simulink model "sampleModel646original"  (R2021b)
settings: Solver=VariableStepAuto  StartTime=0.0  StopTime=10.0  RelTol=1e-3
undefined symbols (not defined in the file): DiscIntNeverNeededParam, Newton, Raphson, sigbuilder_block
libraries: simulink x194, slpidlib x27
(part 2 of 5)

== system sampleModel646original/emi_1101 ==
  In1 : Inport
  emi_1102 : Inport  Port=2
  emi_1104 : Sin  TimeSource=Use external signal  SampleTime=0
  emi_1105 : simulink/Discrete/Difference  ICPrevInput=0.0  OutMin=[]  OutMax=[]  OutDataType=fixdt(1, 16)  OutScaling=2^-10  DoSatur=off
  emi_1106 : Sqrt  Operator=rSqrt  SaturateOnIntegerOverflow=on
  emi_1107 : DiscreteStateSpace  SampleTime=-1
  emi_1108 : Sin  TimeSource=Use external signal  SampleTime=0
  emi_1109 : RateLimiter  SampleTimeMode=inherited
  emi_1110 : Sin  TimeSource=Use external signal  SampleTime=0
  emi_1111 : slpidlib/PID Controller  Controller=PID  Form=Parallel  TimeDomain=Discrete-time  UseExternalTs=off  SampleTime=-1  IntegratorMethod=Forward Euler  FilterMethod=Forward Euler  ControllerParametersSource=internal  P=1  I=1  D=0  UseFilter=on  N=100  TunerSelectOption=Transfer Function Based (PID Tuner App)  InitialConditionSource=internal  InitialConditionForIntegrator=0  InitialConditionForFilter=0  DifferentiatorICPrevScaledInput=0  ExternalReset=none  TrackingMode=off  Kt=1  LimitOutput=off  SatLimitsSource=internal  UpperSaturationLimit=inf  LowerSaturationLimit=-inf  LinearizeAsGain=off  AntiWindupMode=none  Kb=1  POutMin=[]  POutMax=[]  IOutMin=[]  IOutMax=[]  DOutMin=[]  DOutMax=[]  NOutMin=[]  NOutMax=[]  SumOutMin=[]  SumOutMax=[]  SaturationOutMin=[]  SaturationOutMax=[]  PParamMin=[]  PParamMax=[]  IParamMin=[]  IParamMax=[]  DParamMin=[]  DParamMax=[]  NParamMin=[]  NParamMax=[]  KbParamMin=[]  KbParamMax=[]  KtParamMin=[]  KtParamMax=[]  KbOutMin=[]  KbOutMax=[]  KtOutMin=[]  KtOutMax=[]  IntegratorOutMin=[]  IntegratorOutMax=[]  FilterOutMin=[]  FilterOutMax=[]  SumI1OutMin=[]  SumI1OutMax=[]  SumI2OutMin=[]  SumI2OutMax=[]  SumI3OutMin=[]  SumI3OutMax=[]  SumI4OutMin=[]  SumI4OutMax=[]  SumDOutMin=[]  SumDOutMax=[]  DifferentiatorOutMin=[]  DifferentiatorOutMax=[]  FilterDiffOutCoefMin=[]  FilterDiffOutCoefMax=[]  ReciprocalOutMin=[]  ReciprocalOutMax=[]  SumDenOutMin=[]  SumDenOutMax=[]  SumNumOutMin=[]  SumNumOutMax=[]  DivideOutMin=[]  DivideOutMax=[]  UdiffTsProdOutMin=[]  UdiffTsProdOutMax=[]  NTsProdOutMin=[]  NTsProdOutMax=[]  UintegralTsProdOutMin=[]  UintegralTsProdOutMax=[]  UngainTsProdOutMin=[]  UngainTsProdOutMax=[]  IntegratorContinuousStateAttributes=''  IntegratorStateMustResolveToSignalObject=off  IntegratorRTWStateStorageClass=Auto  FilterContinuousStateAttributes=''  FilterStateMustResolveToSignalObject=off  FilterRTWStateStorageClass=Auto  ParallelPVariant=InternalParameters  IdealPVariant=Disabled  IVariant=InternalParameters  DVariant=InternalParameters  IntegratorVariant=Discrete  SatVariant=Disabled  AWVariant=Passthrough  PCopyVariant=Disabled  TRVariant=Disabled  FdbkBlocksVariant=Forward  IdealPFdbkVariant=Disabled  SatFdbkVariant=Disabled  DerivativeFilterVariant=ForwardEulerFilter  NVariant=InternalParameters  NCopyVariant=Disabled  FilterICVariant=InternalICsFilter  IntegratorICVariant=InternalICs  ExternalResetVariant=Disabled  TRSumVariant=Passthrough  SumFdbkVariant=Disabled  SumVariant=Sum_PID  TsampFilterVariant=InternalTs  TsampNgainVariant=Passthrough  TsampIntegralVariant=Passthrough  ExternalSaturationOutDataTypeStr=Inherit: Same as second input
  emi_1112 : DiscreteFilter
  emi_1113 : simulink/Discrete/Transfer Fcn First Order  PoleZ=0.95  ICPrevOutput=0.0  DoSatur=off
  emi_1114 : Math  SaturateOnIntegerOverflow=on
  emi_1115 : DeadZone  SaturateOnIntegerOverflow=on
  emi_1116 : DiscreteTransferFcn
  emi_1117 : simulink/Sources/Chirp Signal  f1=0.1  T=100  f2=1
  Out1 : Outport
  emi_1103 : Outport  Port=2
  wires:
  In1/1 -> Out1/1
  emi_1104/1 -> emi_1105/1
  emi_1105/1 -> emi_1106/1
  emi_1106/1 -> emi_1107/1
  emi_1107/1 -> emi_1108/1
  emi_1108/1 -> emi_1109/1
  emi_1109/1 -> emi_1110/1
  emi_1110/1 -> emi_1111/1
  emi_1111/1 -> emi_1112/1
  emi_1112/1 -> emi_1113/1
  emi_1113/1 -> emi_1114/1
  emi_1114/1 -> emi_1115/1
  emi_1115/1 -> emi_1116/1
  emi_1117/1 -> emi_1104/1
  emi_1116/1 -> emi_1103/1

== system sampleModel646original/emi_1124 ==
  emi_1131 : Inport
  Action Port : ActionPort  ActionPortLabel=if(-1.382844e+09 > u1)
  emi_{1128..1129,1136,1138} (4 alike) : Math  SaturateOnIntegerOverflow=on
  emi_1130 : MinMax
  emi_{1133..1135,1143} (4 alike) : Sin  TimeSource=Use external signal  SampleTime=0
  emi_{1137,1139..1140,1142} (4 alike) : UnaryMinus
  emi_1141 : Sqrt  Operator=rSqrt  SaturateOnIntegerOverflow=on
  emi_1144 : Product  Inputs=*
  emi_1145 : Ground
  emi_1132 : Outport
  wires:
  emi_1131/1 -> emi_1128/1
  emi_1128/1 -> emi_1129/1
  emi_1129/1 -> emi_1130/1
  emi_1133/1 -> emi_1134/1
  emi_1134/1 -> emi_1135/1
  emi_1135/1 -> emi_1136/1
  emi_1136/1 -> emi_1137/1
  emi_1137/1 -> emi_1138/1
  emi_1138/1 -> emi_1139/1
  emi_1139/1 -> emi_1140/1
  emi_1140/1 -> emi_1141/1
  emi_1141/1 -> emi_1142/1
  emi_1142/1 -> emi_1143/1
  emi_1143/1 -> emi_1144/1
  emi_1145/1 -> emi_1133/1
  emi_1144/1 -> emi_1132/1

== system sampleModel646original/emi_1148 ==
  In1 : Inport
  emi_1149 : Inport  Port=2
  emi_1151 : simulink/Discrete/Difference  ICPrevInput=0.0  OutMin=[]  OutMax=[]  OutDataType=fixdt(1, 16)  OutScaling=2^-10  DoSatur=off
  emi_1152 : simulink/Discrete/Transfer Fcn First Order  PoleZ=0.95  ICPrevOutput=0.0  DoSatur=off
  emi_1153 : DiscreteZeroPole  Poles=[0 0.5]  Gain=1  SampleTime=-1
  emi_1154 : RateLimiter  SampleTimeMode=inherited
  emi_1155 : DeadZone  SaturateOnIntegerOverflow=on
  emi_1156 : Rounding
  emi_1157 : simulink/Discrete/Discrete Derivative  gainval=1.0  ICPrevScaledInput=0.0  OutMin=[]  OutMax=[]  OutDataType=fixdt(1, 16)  OutScaling=2^-10  DoSatur=off
  emi_1158 : VariablePulseGenerator  SampleTime=0.1
  emi_1159 : Gain
  emi_1160 : Sum  Inputs=+
  emi_1161 : simulink/Sources/Repeating Sequence Interpolated  OutValues=[3 1 4 2 1].'  TimeValues=[0 0.1 0.5 0.6 1].'  LookUpMeth=Interpolation-Use End Values  tsamp=0.01  OutMin=[]  OutMax=[]  OutDataTypeStr=double  OutputDataTypeScalingMode=double  OutDataType=fixdt(0,8)  OutScaling=2^-10
  Out1 : Outport
  emi_1150 : Outport  Port=2
  wires:
  In1/1 -> Out1/1
  emi_1151/1 -> emi_1152/1
  emi_1152/1 -> emi_1153/1
  emi_1153/1 -> emi_1154/1
  emi_1154/1 -> emi_1155/1
  emi_1155/1 -> emi_1156/1
  emi_1156/1 -> emi_1157/1
  emi_1157/1 -> emi_1158/1
  emi_1158/1 -> emi_1159/1
  emi_1159/1 -> emi_1160/1
  emi_1161/1 -> emi_1151/1
  emi_1160/1 -> emi_1150/1

== system sampleModel646original/emi_1168 ==
  emi_1175 : Inport
  Action Port : ActionPort  ActionPortLabel=if(0 > u1)
  emi_1172 : Gain
  emi_1173 : MinMax
  emi_{1174,1180..1181,1195..1197} (6 alike) : Math  SaturateOnIntegerOverflow=on
  emi_{1177,1182,1192,1202} (4 alike) : Sin  TimeSource=Use external signal  SampleTime=0
  emi_1178 : Trigonometry
  emi_1179 : Sqrt  Operator=rSqrt  SaturateOnIntegerOverflow=on
  emi_{1183,1190,1198,1200..1201} (5 alike) : Rounding
  emi_1184 : UnaryMinus
  emi_1185 : Trigonometry
  emi_{1186,1188..1189,1193} (4 alike) : Sum  Inputs=+
  emi_1187 : Product  Inputs=*
  emi_1191 : MinMax
  emi_1194 : Abs
  emi_1199 : MinMax
  emi_1203 : Ground
  emi_1176 : Outport
  wires:
  emi_1175/1 -> emi_1172/1
  emi_1172/1 -> emi_1173/1
  emi_1173/1 -> emi_1174/1
  emi_1177/1 -> emi_1178/1
  emi_1178/1 -> emi_1179/1
  emi_1179/1 -> emi_1180/1
  emi_1180/1 -> emi_1181/1
  emi_1181/1 -> emi_1182/1
  emi_1182/1 -> emi_1183/1
  emi_1183/1 -> emi_1184/1
  emi_1184/1 -> emi_1185/1
  emi_1185/1 -> emi_1186/1
  emi_1186/1 -> emi_1187/1
  emi_1187/1 -> emi_1188/1
  emi_1188/1 -> emi_1189/1
  emi_1189/1 -> emi_1190/1
  emi_1190/1 -> emi_1191/1
  emi_1191/1 -> emi_1192/1
  emi_1192/1 -> emi_1193/1
  emi_1193/1 -> emi_1194/1
  emi_1194/1 -> emi_1195/1
  emi_1195/1 -> emi_1196/1
  emi_1196/1 -> emi_1197/1
  emi_1197/1 -> emi_1198/1
  emi_1198/1 -> emi_1199/1
  emi_1199/1 -> emi_1200/1
  emi_1200/1 -> emi_1201/1
  emi_1201/1 -> emi_1202/1
  emi_1203/1 -> emi_1177/1
  emi_1202/1 -> emi_1176/1

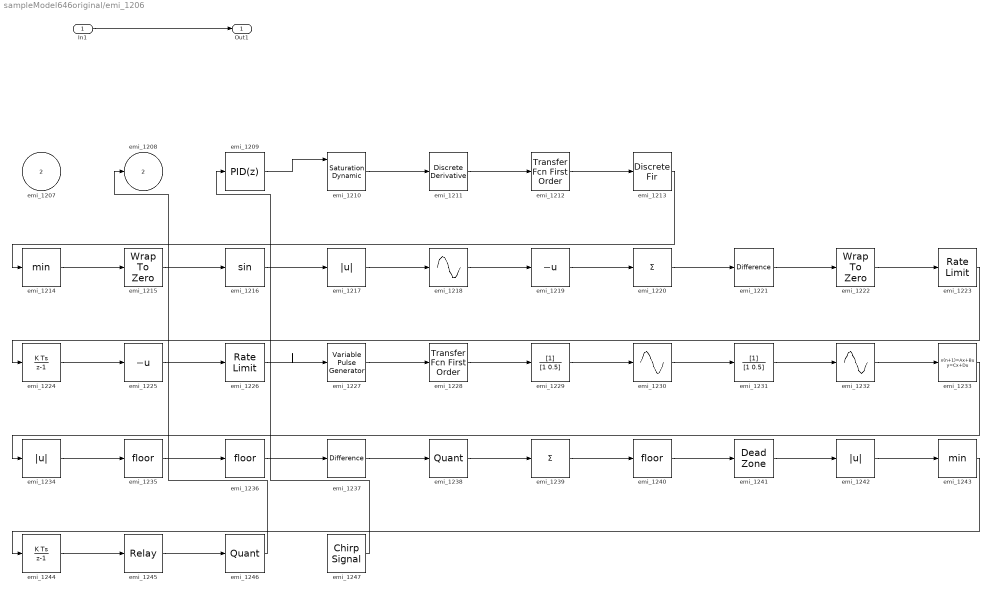
== system sampleModel646original/emi_1206 ==
  In1 : Inport
  emi_1207 : Inport  Port=2
  emi_1209 : slpidlib/PID Controller  Controller=PID  Form=Parallel  TimeDomain=Discrete-time  UseExternalTs=off  SampleTime=-1  IntegratorMethod=Forward Euler  FilterMethod=Forward Euler  ControllerParametersSource=internal  P=1  I=1  D=0  UseFilter=on  N=100  TunerSelectOption=Transfer Function Based (PID Tuner App)  InitialConditionSource=internal  InitialConditionForIntegrator=0  InitialConditionForFilter=0  DifferentiatorICPrevScaledInput=0  ExternalReset=none  TrackingMode=off  Kt=1  LimitOutput=off  SatLimitsSource=internal  UpperSaturationLimit=inf  LowerSaturationLimit=-inf  LinearizeAsGain=off  AntiWindupMode=none  Kb=1  POutMin=[]  POutMax=[]  IOutMin=[]  IOutMax=[]  DOutMin=[]  DOutMax=[]  NOutMin=[]  NOutMax=[]  SumOutMin=[]  SumOutMax=[]  SaturationOutMin=[]  SaturationOutMax=[]  PParamMin=[]  PParamMax=[]  IParamMin=[]  IParamMax=[]  DParamMin=[]  DParamMax=[]  NParamMin=[]  NParamMax=[]  KbParamMin=[]  KbParamMax=[]  KtParamMin=[]  KtParamMax=[]  KbOutMin=[]  KbOutMax=[]  KtOutMin=[]  KtOutMax=[]  IntegratorOutMin=[]  IntegratorOutMax=[]  FilterOutMin=[]  FilterOutMax=[]  SumI1OutMin=[]  SumI1OutMax=[]  SumI2OutMin=[]  SumI2OutMax=[]  SumI3OutMin=[]  SumI3OutMax=[]  SumI4OutMin=[]  SumI4OutMax=[]  SumDOutMin=[]  SumDOutMax=[]  DifferentiatorOutMin=[]  DifferentiatorOutMax=[]  FilterDiffOutCoefMin=[]  FilterDiffOutCoefMax=[]  ReciprocalOutMin=[]  ReciprocalOutMax=[]  SumDenOutMin=[]  SumDenOutMax=[]  SumNumOutMin=[]  SumNumOutMax=[]  DivideOutMin=[]  DivideOutMax=[]  UdiffTsProdOutMin=[]  UdiffTsProdOutMax=[]  NTsProdOutMin=[]  NTsProdOutMax=[]  UintegralTsProdOutMin=[]  UintegralTsProdOutMax=[]  UngainTsProdOutMin=[]  UngainTsProdOutMax=[]  IntegratorContinuousStateAttributes=''  IntegratorStateMustResolveToSignalObject=off  IntegratorRTWStateStorageClass=Auto  FilterContinuousStateAttributes=''  FilterStateMustResolveToSignalObject=off  FilterRTWStateStorageClass=Auto  ParallelPVariant=InternalParameters  IdealPVariant=Disabled  IVariant=InternalParameters  DVariant=InternalParameters  IntegratorVariant=Discrete  SatVariant=Disabled  AWVariant=Passthrough  PCopyVariant=Disabled  TRVariant=Disabled  FdbkBlocksVariant=Forward  IdealPFdbkVariant=Disabled  SatFdbkVariant=Disabled  DerivativeFilterVariant=ForwardEulerFilter  NVariant=InternalParameters  NCopyVariant=Disabled  FilterICVariant=InternalICsFilter  IntegratorICVariant=InternalICs  ExternalResetVariant=Disabled  TRSumVariant=Passthrough  SumFdbkVariant=Disabled  SumVariant=Sum_PID  TsampFilterVariant=InternalTs  TsampNgainVariant=Passthrough  TsampIntegralVariant=Passthrough  ExternalSaturationOutDataTypeStr=Inherit: Same as second input
  emi_1210 : simulink/Discontinuities/Saturation Dynamic  OutMin=[]  OutMax=[]  OutDataTypeStr=Inherit: Same as second input  OutDataType=fixdt(1, 16)  OutScaling=2^-10  DoSatur=off
  emi_1211 : simulink/Discrete/Discrete Derivative  gainval=1.0  ICPrevScaledInput=0.0  OutMin=[]  OutMax=[]  OutDataType=fixdt(1, 16)  OutScaling=2^-10  DoSatur=off
  emi_1212 : simulink/Discrete/Transfer Fcn First Order  PoleZ=0.95  ICPrevOutput=0.0  DoSatur=off
  emi_1213 : DiscreteFir
  emi_1214 : MinMax
  emi_1215 : simulink/Discontinuities/Wrap To Zero  Threshold=255
      settings: SourceProductBaseCode=SL
  emi_1216 : Trigonometry
  emi_1217 : Abs
  emi_1218 : Sin  TimeSource=Use external signal  SampleTime=0
  emi_1219 : UnaryMinus
  emi_1220 : Sum  Inputs=+
  emi_1221 : simulink/Discrete/Difference  ICPrevInput=0.0  OutMin=[]  OutMax=[]  OutDataType=fixdt(1, 16)  OutScaling=2^-10  DoSatur=off
  emi_1222 : simulink/Discontinuities/Wrap To Zero  Threshold=255
      settings: SourceProductBaseCode=SL
  emi_1223 : RateLimiter  SampleTimeMode=inherited
  emi_1224 : DiscreteIntegrator  SampleTime=-1  ICPrevOutput=DiscIntNeverNeededParam  ICPrevScaledInput=DiscIntNeverNeededParam
  emi_1225 : UnaryMinus
  emi_1226 : RateLimiter  SampleTimeMode=inherited
  emi_1227 : VariablePulseGenerator  SampleTime=0.1
  emi_1228 : simulink/Discrete/Transfer Fcn First Order  PoleZ=0.95  ICPrevOutput=0.0  DoSatur=off
  emi_1229 : DiscreteFilter
  emi_1230 : Sin  TimeSource=Use external signal  SampleTime=0
  emi_1231 : DiscreteFilter
  emi_1232 : Sin  TimeSource=Use external signal  SampleTime=0
  emi_1233 : DiscreteStateSpace  SampleTime=-1
  emi_1234 : Abs
  emi_1235 : Rounding
  emi_1236 : Rounding
  emi_1237 : simulink/Discrete/Difference  ICPrevInput=0.0  OutMin=[]  OutMax=[]  OutDataType=fixdt(1, 16)  OutScaling=2^-10  DoSatur=off
  emi_1238 : Quantizer
  emi_1239 : Sum  Inputs=+
  emi_1240 : Rounding
  emi_1241 : DeadZone  SaturateOnIntegerOverflow=on
  emi_1242 : Abs
  emi_1243 : MinMax
  emi_1244 : DiscreteIntegrator  SampleTime=-1  ICPrevOutput=DiscIntNeverNeededParam  ICPrevScaledInput=DiscIntNeverNeededParam
  emi_1245 : Relay
  emi_1246 : Quantizer
  emi_1247 : simulink/Sources/Chirp Signal  f1=0.1  T=100  f2=1
  Out1 : Outport
  emi_1208 : Outport  Port=2
  wires:
  In1/1 -> Out1/1
  emi_1209/1 -> emi_1210/1
  emi_1210/1 -> emi_1211/1
  emi_1211/1 -> emi_1212/1
  emi_1212/1 -> emi_1213/1
  emi_1213/1 -> emi_1214/1
  emi_1214/1 -> emi_1215/1
  emi_1215/1 -> emi_1216/1
  emi_1216/1 -> emi_1217/1
  emi_1217/1 -> emi_1218/1
  emi_1218/1 -> emi_1219/1
  emi_1219/1 -> emi_1220/1
  emi_1220/1 -> emi_1221/1
  emi_1221/1 -> emi_1222/1
  emi_1222/1 -> emi_1223/1
  emi_1223/1 -> emi_1224/1
  emi_1224/1 -> emi_1225/1
  emi_1225/1 -> emi_1226/1
  emi_1226/1 -> emi_1227/1
  emi_1227/1 -> emi_1228/1
  emi_1228/1 -> emi_1229/1
  emi_1229/1 -> emi_1230/1
  emi_1230/1 -> emi_1231/1
  emi_1231/1 -> emi_1232/1
  emi_1232/1 -> emi_1233/1
  emi_1233/1 -> emi_1234/1
  emi_1234/1 -> emi_1235/1
  emi_1235/1 -> emi_1236/1
  emi_1236/1 -> emi_1237/1
  emi_1237/1 -> emi_1238/1
  emi_1238/1 -> emi_1239/1
  emi_1239/1 -> emi_1240/1
  emi_1240/1 -> emi_1241/1
  emi_1241/1 -> emi_1242/1
  emi_1242/1 -> emi_1243/1
  emi_1243/1 -> emi_1244/1
  emi_1244/1 -> emi_1245/1
  emi_1245/1 -> emi_1246/1
  emi_1247/1 -> emi_1209/1
  emi_1246/1 -> emi_1208/1

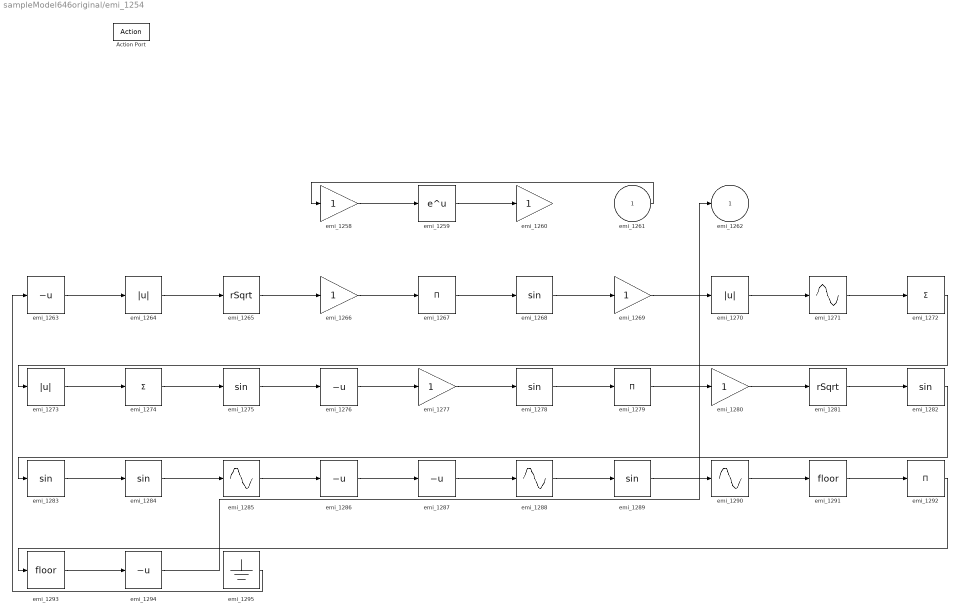
== system sampleModel646original/emi_1254 ==
  emi_1261 : Inport
  Action Port : ActionPort  ActionPortLabel=if(0 > u1)
  emi_{1258,1260,1266,1269,1277,1280} (6 alike) : Gain
  emi_1259 : Math  SaturateOnIntegerOverflow=on
  emi_{1263,1276,1286..1287,1294} (5 alike) : UnaryMinus
  emi_1264 : Abs
  emi_1265 : Sqrt  Operator=rSqrt  SaturateOnIntegerOverflow=on
  emi_1267 : Product  Inputs=*
  emi_{1268,1275,1278,1282..1284,1289} (7 alike) : Trigonometry
  emi_1270 : Abs
  emi_{1271,1285,1288,1290} (4 alike) : Sin  TimeSource=Use external signal  SampleTime=0
  emi_1272 : Sum  Inputs=+
  emi_1273 : Abs
  emi_1274 : Sum  Inputs=+
  emi_1279 : Product  Inputs=*
  emi_1281 : Sqrt  Operator=rSqrt  SaturateOnIntegerOverflow=on
  emi_1291 : Rounding
  emi_1292 : Product  Inputs=*
  emi_1293 : Rounding
  emi_1295 : Ground
  emi_1262 : Outport
  wires:
  emi_1261/1 -> emi_1258/1
  emi_1258/1 -> emi_1259/1
  emi_1259/1 -> emi_1260/1
  emi_1263/1 -> emi_1264/1
  emi_1264/1 -> emi_1265/1
  emi_1265/1 -> emi_1266/1
  emi_1266/1 -> emi_1267/1
  emi_1267/1 -> emi_1268/1
  emi_1268/1 -> emi_1269/1
  emi_1269/1 -> emi_1270/1
  emi_1270/1 -> emi_1271/1
  emi_1271/1 -> emi_1272/1
  emi_1272/1 -> emi_1273/1
  emi_1273/1 -> emi_1274/1
  emi_1274/1 -> emi_1275/1
  emi_1275/1 -> emi_1276/1
  emi_1276/1 -> emi_1277/1
  emi_1277/1 -> emi_1278/1
  emi_1278/1 -> emi_1279/1
  emi_1279/1 -> emi_1280/1
  emi_1280/1 -> emi_1281/1
  emi_1281/1 -> emi_1282/1
  emi_1282/1 -> emi_1283/1
  emi_1283/1 -> emi_1284/1
  emi_1284/1 -> emi_1285/1
  emi_1285/1 -> emi_1286/1
  emi_1286/1 -> emi_1287/1
  emi_1287/1 -> emi_1288/1
  emi_1288/1 -> emi_1289/1
  emi_1289/1 -> emi_1290/1
  emi_1290/1 -> emi_1291/1
  emi_1291/1 -> emi_1292/1
  emi_1292/1 -> emi_1293/1
  emi_1293/1 -> emi_1294/1
  emi_1295/1 -> emi_1263/1
  emi_1294/1 -> emi_1262/1

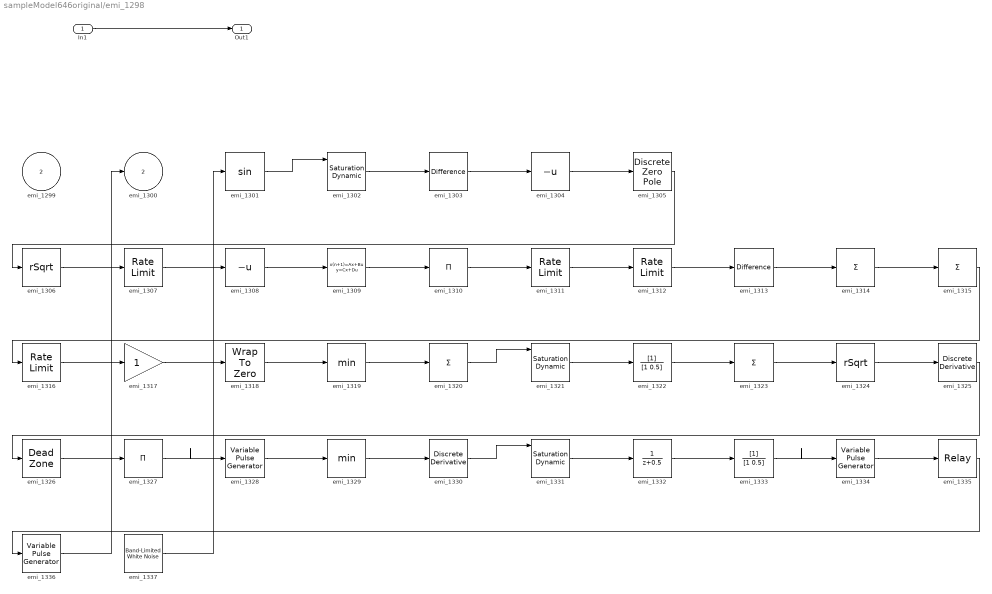
== system sampleModel646original/emi_1298 ==
  In1 : Inport
  emi_1299 : Inport  Port=2
  emi_1301 : Trigonometry
  emi_1302 : simulink/Discontinuities/Saturation Dynamic  OutMin=[]  OutMax=[]  OutDataTypeStr=Inherit: Same as second input  OutDataType=fixdt(1, 16)  OutScaling=2^-10  DoSatur=off
  emi_1303 : simulink/Discrete/Difference  ICPrevInput=0.0  OutMin=[]  OutMax=[]  OutDataType=fixdt(1, 16)  OutScaling=2^-10  DoSatur=off
  emi_1304 : UnaryMinus
  emi_1305 : DiscreteZeroPole  Poles=[0 0.5]  Gain=1  SampleTime=-1
  emi_1306 : Sqrt  Operator=rSqrt  SaturateOnIntegerOverflow=on
  emi_{1307,1311..1312,1316} (4 alike) : RateLimiter  SampleTimeMode=inherited
  emi_1308 : UnaryMinus
  emi_1309 : DiscreteStateSpace  SampleTime=-1
  emi_1310 : Product  Inputs=*
  emi_1313 : simulink/Discrete/Difference  ICPrevInput=0.0  OutMin=[]  OutMax=[]  OutDataType=fixdt(1, 16)  OutScaling=2^-10  DoSatur=off
  emi_{1314..1315,1320,1323} (4 alike) : Sum  Inputs=+
  emi_1317 : Gain
  emi_1318 : simulink/Discontinuities/Wrap To Zero  Threshold=255
      settings: SourceProductBaseCode=SL
  emi_1319 : MinMax
  emi_1321 : simulink/Discontinuities/Saturation Dynamic  OutMin=[]  OutMax=[]  OutDataTypeStr=Inherit: Same as second input  OutDataType=fixdt(1, 16)  OutScaling=2^-10  DoSatur=off
  emi_1322 : DiscreteFilter
  emi_1324 : Sqrt  Operator=rSqrt  SaturateOnIntegerOverflow=on
  emi_1325 : simulink/Discrete/Discrete Derivative  gainval=1.0  ICPrevScaledInput=0.0  OutMin=[]  OutMax=[]  OutDataType=fixdt(1, 16)  OutScaling=2^-10  DoSatur=off
  emi_1326 : DeadZone  SaturateOnIntegerOverflow=on
  emi_1327 : Product  Inputs=*
  emi_1328 : VariablePulseGenerator  SampleTime=0.1
  emi_1329 : MinMax
  emi_1330 : simulink/Discrete/Discrete Derivative  gainval=1.0  ICPrevScaledInput=0.0  OutMin=[]  OutMax=[]  OutDataType=fixdt(1, 16)  OutScaling=2^-10  DoSatur=off
  emi_1331 : simulink/Discontinuities/Saturation Dynamic  OutMin=[]  OutMax=[]  OutDataTypeStr=Inherit: Same as second input  OutDataType=fixdt(1, 16)  OutScaling=2^-10  DoSatur=off
  emi_1332 : DiscreteTransferFcn
  emi_1333 : DiscreteFilter
  emi_1334 : VariablePulseGenerator  SampleTime=0.1
  emi_1335 : Relay
  emi_1336 : VariablePulseGenerator  SampleTime=0.1
  emi_1337 : simulink/Sources/Band-Limited White Noise  Cov=[0.1]  Ts=0.1  seed=[23341]
  Out1 : Outport
  emi_1300 : Outport  Port=2
  wires:
  In1/1 -> Out1/1
  emi_1301/1 -> emi_1302/1
  emi_1302/1 -> emi_1303/1
  emi_1303/1 -> emi_1304/1
  emi_1304/1 -> emi_1305/1
  emi_1305/1 -> emi_1306/1
  emi_1306/1 -> emi_1307/1
  emi_1307/1 -> emi_1308/1
  emi_1308/1 -> emi_1309/1
  emi_1309/1 -> emi_1310/1
  emi_1310/1 -> emi_1311/1
  emi_1311/1 -> emi_1312/1
  emi_1312/1 -> emi_1313/1
  emi_1313/1 -> emi_1314/1
  emi_1314/1 -> emi_1315/1
  emi_1315/1 -> emi_1316/1
  emi_1316/1 -> emi_1317/1
  emi_1317/1 -> emi_1318/1
  emi_1318/1 -> emi_1319/1
  emi_1319/1 -> emi_1320/1
  emi_1320/1 -> emi_1321/1
  emi_1321/1 -> emi_1322/1
  emi_1322/1 -> emi_1323/1
  emi_1323/1 -> emi_1324/1
  emi_1324/1 -> emi_1325/1
  emi_1325/1 -> emi_1326/1
  emi_1326/1 -> emi_1327/1
  emi_1327/1 -> emi_1328/1
  emi_1328/1 -> emi_1329/1
  emi_1329/1 -> emi_1330/1
  emi_1330/1 -> emi_1331/1
  emi_1331/1 -> emi_1332/1
  emi_1332/1 -> emi_1333/1
  emi_1333/1 -> emi_1334/1
  emi_1334/1 -> emi_1335/1
  emi_1335/1 -> emi_1336/1
  emi_1337/1 -> emi_1301/1
  emi_1336/1 -> emi_1300/1

== system sampleModel646original/emi_132 ==
  In1 : Inport
  emi_133 : Inport  Port=2
  emi_135 : DiscreteStateSpace  SampleTime=-1
  emi_136 : slpidlib/PID Controller  Controller=PID  Form=Parallel  TimeDomain=Discrete-time  UseExternalTs=off  SampleTime=-1  IntegratorMethod=Forward Euler  FilterMethod=Forward Euler  ControllerParametersSource=internal  P=1  I=1  D=0  UseFilter=on  N=100  TunerSelectOption=Transfer Function Based (PID Tuner App)  InitialConditionSource=internal  InitialConditionForIntegrator=0  InitialConditionForFilter=0  DifferentiatorICPrevScaledInput=0  ExternalReset=none  TrackingMode=off  Kt=1  LimitOutput=off  SatLimitsSource=internal  UpperSaturationLimit=inf  LowerSaturationLimit=-inf  LinearizeAsGain=off  AntiWindupMode=none  Kb=1  POutMin=[]  POutMax=[]  IOutMin=[]  IOutMax=[]  DOutMin=[]  DOutMax=[]  NOutMin=[]  NOutMax=[]  SumOutMin=[]  SumOutMax=[]  SaturationOutMin=[]  SaturationOutMax=[]  PParamMin=[]  PParamMax=[]  IParamMin=[]  IParamMax=[]  DParamMin=[]  DParamMax=[]  NParamMin=[]  NParamMax=[]  KbParamMin=[]  KbParamMax=[]  KtParamMin=[]  KtParamMax=[]  KbOutMin=[]  KbOutMax=[]  KtOutMin=[]  KtOutMax=[]  IntegratorOutMin=[]  IntegratorOutMax=[]  FilterOutMin=[]  FilterOutMax=[]  SumI1OutMin=[]  SumI1OutMax=[]  SumI2OutMin=[]  SumI2OutMax=[]  SumI3OutMin=[]  SumI3OutMax=[]  SumI4OutMin=[]  SumI4OutMax=[]  SumDOutMin=[]  SumDOutMax=[]  DifferentiatorOutMin=[]  DifferentiatorOutMax=[]  FilterDiffOutCoefMin=[]  FilterDiffOutCoefMax=[]  ReciprocalOutMin=[]  ReciprocalOutMax=[]  SumDenOutMin=[]  SumDenOutMax=[]  SumNumOutMin=[]  SumNumOutMax=[]  DivideOutMin=[]  DivideOutMax=[]  UdiffTsProdOutMin=[]  UdiffTsProdOutMax=[]  NTsProdOutMin=[]  NTsProdOutMax=[]  UintegralTsProdOutMin=[]  UintegralTsProdOutMax=[]  UngainTsProdOutMin=[]  UngainTsProdOutMax=[]  IntegratorContinuousStateAttributes=''  IntegratorStateMustResolveToSignalObject=off  IntegratorRTWStateStorageClass=Auto  FilterContinuousStateAttributes=''  FilterStateMustResolveToSignalObject=off  FilterRTWStateStorageClass=Auto  ParallelPVariant=InternalParameters  IdealPVariant=Disabled  IVariant=InternalParameters  DVariant=InternalParameters  IntegratorVariant=Discrete  SatVariant=Disabled  AWVariant=Passthrough  PCopyVariant=Disabled  TRVariant=Disabled  FdbkBlocksVariant=Forward  IdealPFdbkVariant=Disabled  SatFdbkVariant=Disabled  DerivativeFilterVariant=ForwardEulerFilter  NVariant=InternalParameters  NCopyVariant=Disabled  FilterICVariant=InternalICsFilter  IntegratorICVariant=InternalICs  ExternalResetVariant=Disabled  TRSumVariant=Passthrough  SumFdbkVariant=Disabled  SumVariant=Sum_PID  TsampFilterVariant=InternalTs  TsampNgainVariant=Passthrough  TsampIntegralVariant=Passthrough  ExternalSaturationOutDataTypeStr=Inherit: Same as second input
  emi_137 : Math  SaturateOnIntegerOverflow=on
  emi_138 : Sum  Inputs=+
  emi_139 : slpidlib/PID Controller  Controller=PID  Form=Parallel  TimeDomain=Discrete-time  UseExternalTs=off  SampleTime=-1  IntegratorMethod=Forward Euler  FilterMethod=Forward Euler  ControllerParametersSource=internal  P=1  I=1  D=0  UseFilter=on  N=100  TunerSelectOption=Transfer Function Based (PID Tuner App)  InitialConditionSource=internal  InitialConditionForIntegrator=0  InitialConditionForFilter=0  DifferentiatorICPrevScaledInput=0  ExternalReset=none  TrackingMode=off  Kt=1  LimitOutput=off  SatLimitsSource=internal  UpperSaturationLimit=inf  LowerSaturationLimit=-inf  LinearizeAsGain=off  AntiWindupMode=none  Kb=1  POutMin=[]  POutMax=[]  IOutMin=[]  IOutMax=[]  DOutMin=[]  DOutMax=[]  NOutMin=[]  NOutMax=[]  SumOutMin=[]  SumOutMax=[]  SaturationOutMin=[]  SaturationOutMax=[]  PParamMin=[]  PParamMax=[]  IParamMin=[]  IParamMax=[]  DParamMin=[]  DParamMax=[]  NParamMin=[]  NParamMax=[]  KbParamMin=[]  KbParamMax=[]  KtParamMin=[]  KtParamMax=[]  KbOutMin=[]  KbOutMax=[]  KtOutMin=[]  KtOutMax=[]  IntegratorOutMin=[]  IntegratorOutMax=[]  FilterOutMin=[]  FilterOutMax=[]  SumI1OutMin=[]  SumI1OutMax=[]  SumI2OutMin=[]  SumI2OutMax=[]  SumI3OutMin=[]  SumI3OutMax=[]  SumI4OutMin=[]  SumI4OutMax=[]  SumDOutMin=[]  SumDOutMax=[]  DifferentiatorOutMin=[]  DifferentiatorOutMax=[]  FilterDiffOutCoefMin=[]  FilterDiffOutCoefMax=[]  ReciprocalOutMin=[]  ReciprocalOutMax=[]  SumDenOutMin=[]  SumDenOutMax=[]  SumNumOutMin=[]  SumNumOutMax=[]  DivideOutMin=[]  DivideOutMax=[]  UdiffTsProdOutMin=[]  UdiffTsProdOutMax=[]  NTsProdOutMin=[]  NTsProdOutMax=[]  UintegralTsProdOutMin=[]  UintegralTsProdOutMax=[]  UngainTsProdOutMin=[]  UngainTsProdOutMax=[]  IntegratorContinuousStateAttributes=''  IntegratorStateMustResolveToSignalObject=off  IntegratorRTWStateStorageClass=Auto  FilterContinuousStateAttributes=''  FilterStateMustResolveToSignalObject=off  FilterRTWStateStorageClass=Auto  ParallelPVariant=InternalParameters  IdealPVariant=Disabled  IVariant=InternalParameters  DVariant=InternalParameters  IntegratorVariant=Discrete  SatVariant=Disabled  AWVariant=Passthrough  PCopyVariant=Disabled  TRVariant=Disabled  FdbkBlocksVariant=Forward  IdealPFdbkVariant=Disabled  SatFdbkVariant=Disabled  DerivativeFilterVariant=ForwardEulerFilter  NVariant=InternalParameters  NCopyVariant=Disabled  FilterICVariant=InternalICsFilter  IntegratorICVariant=InternalICs  ExternalResetVariant=Disabled  TRSumVariant=Passthrough  SumFdbkVariant=Disabled  SumVariant=Sum_PID  TsampFilterVariant=InternalTs  TsampNgainVariant=Passthrough  TsampIntegralVariant=Passthrough  ExternalSaturationOutDataTypeStr=Inherit: Same as second input
  emi_140 : RateLimiter  SampleTimeMode=inherited
  emi_141 : Gain
  emi_142 : Sqrt  Operator=rSqrt  SaturateOnIntegerOverflow=on
  emi_143 : DeadZone  SaturateOnIntegerOverflow=on
  emi_144 : Relay
  emi_145 : Quantizer
  emi_146 : DiscreteIntegrator  SampleTime=-1  ICPrevOutput=DiscIntNeverNeededParam  ICPrevScaledInput=DiscIntNeverNeededParam
  emi_147 : UnaryMinus
  emi_148 : simulink/Discrete/Transfer Fcn First Order  PoleZ=0.95  ICPrevOutput=0.0  DoSatur=off
  emi_149 : Trigonometry
  emi_150 : slpidlib/PID Controller  Controller=PID  Form=Parallel  TimeDomain=Discrete-time  UseExternalTs=off  SampleTime=-1  IntegratorMethod=Forward Euler  FilterMethod=Forward Euler  ControllerParametersSource=internal  P=1  I=1  D=0  UseFilter=on  N=100  TunerSelectOption=Transfer Function Based (PID Tuner App)  InitialConditionSource=internal  InitialConditionForIntegrator=0  InitialConditionForFilter=0  DifferentiatorICPrevScaledInput=0  ExternalReset=none  TrackingMode=off  Kt=1  LimitOutput=off  SatLimitsSource=internal  UpperSaturationLimit=inf  LowerSaturationLimit=-inf  LinearizeAsGain=off  AntiWindupMode=none  Kb=1  POutMin=[]  POutMax=[]  IOutMin=[]  IOutMax=[]  DOutMin=[]  DOutMax=[]  NOutMin=[]  NOutMax=[]  SumOutMin=[]  SumOutMax=[]  SaturationOutMin=[]  SaturationOutMax=[]  PParamMin=[]  PParamMax=[]  IParamMin=[]  IParamMax=[]  DParamMin=[]  DParamMax=[]  NParamMin=[]  NParamMax=[]  KbParamMin=[]  KbParamMax=[]  KtParamMin=[]  KtParamMax=[]  KbOutMin=[]  KbOutMax=[]  KtOutMin=[]  KtOutMax=[]  IntegratorOutMin=[]  IntegratorOutMax=[]  FilterOutMin=[]  FilterOutMax=[]  SumI1OutMin=[]  SumI1OutMax=[]  SumI2OutMin=[]  SumI2OutMax=[]  SumI3OutMin=[]  SumI3OutMax=[]  SumI4OutMin=[]  SumI4OutMax=[]  SumDOutMin=[]  SumDOutMax=[]  DifferentiatorOutMin=[]  DifferentiatorOutMax=[]  FilterDiffOutCoefMin=[]  FilterDiffOutCoefMax=[]  ReciprocalOutMin=[]  ReciprocalOutMax=[]  SumDenOutMin=[]  SumDenOutMax=[]  SumNumOutMin=[]  SumNumOutMax=[]  DivideOutMin=[]  DivideOutMax=[]  UdiffTsProdOutMin=[]  UdiffTsProdOutMax=[]  NTsProdOutMin=[]  NTsProdOutMax=[]  UintegralTsProdOutMin=[]  UintegralTsProdOutMax=[]  UngainTsProdOutMin=[]  UngainTsProdOutMax=[]  IntegratorContinuousStateAttributes=''  IntegratorStateMustResolveToSignalObject=off  IntegratorRTWStateStorageClass=Auto  FilterContinuousStateAttributes=''  FilterStateMustResolveToSignalObject=off  FilterRTWStateStorageClass=Auto  ParallelPVariant=InternalParameters  IdealPVariant=Disabled  IVariant=InternalParameters  DVariant=InternalParameters  IntegratorVariant=Discrete  SatVariant=Disabled  AWVariant=Passthrough  PCopyVariant=Disabled  TRVariant=Disabled  FdbkBlocksVariant=Forward  IdealPFdbkVariant=Disabled  SatFdbkVariant=Disabled  DerivativeFilterVariant=ForwardEulerFilter  NVariant=InternalParameters  NCopyVariant=Disabled  FilterICVariant=InternalICsFilter  IntegratorICVariant=InternalICs  ExternalResetVariant=Disabled  TRSumVariant=Passthrough  SumFdbkVariant=Disabled  SumVariant=Sum_PID  TsampFilterVariant=InternalTs  TsampNgainVariant=Passthrough  TsampIntegralVariant=Passthrough  ExternalSaturationOutDataTypeStr=Inherit: Same as second input
  emi_151 : Sqrt  Operator=rSqrt  SaturateOnIntegerOverflow=on
  emi_152 : DiscreteZeroPole  Poles=[0 0.5]  Gain=1  SampleTime=-1
  emi_153 : DeadZone  SaturateOnIntegerOverflow=on
  emi_154 : Sin  TimeSource=Use external signal  SampleTime=0
  emi_155 : DiscreteFilter
  emi_156 : DeadZone  SaturateOnIntegerOverflow=on
  emi_157 : Math  SaturateOnIntegerOverflow=on
  emi_158 : DiscreteIntegrator  SampleTime=-1  ICPrevOutput=DiscIntNeverNeededParam  ICPrevScaledInput=DiscIntNeverNeededParam
  emi_159 : RandomNumber  SampleTime=0.1
  Out1 : Outport
  emi_134 : Outport  Port=2
  wires:
  In1/1 -> Out1/1
  emi_135/1 -> emi_136/1
  emi_136/1 -> emi_137/1
  emi_137/1 -> emi_138/1
  emi_138/1 -> emi_139/1
  emi_139/1 -> emi_140/1
  emi_140/1 -> emi_141/1
  emi_141/1 -> emi_142/1
  emi_142/1 -> emi_143/1
  emi_143/1 -> emi_144/1
  emi_144/1 -> emi_145/1
  emi_145/1 -> emi_146/1
  emi_146/1 -> emi_147/1
  emi_147/1 -> emi_148/1
  emi_148/1 -> emi_149/1
  emi_149/1 -> emi_150/1
  emi_150/1 -> emi_151/1
  emi_151/1 -> emi_152/1
  emi_152/1 -> emi_153/1
  emi_153/1 -> emi_154/1
  emi_154/1 -> emi_155/1
  emi_155/1 -> emi_156/1
  emi_156/1 -> emi_157/1
  emi_157/1 -> emi_158/1
  emi_159/1 -> emi_135/1
  emi_158/1 -> emi_134/1

== system sampleModel646original/emi_1344 ==
  emi_1351 : Inport
  Action Port : ActionPort  ActionPortLabel=if(0 > u1)
  emi_1348 : Trigonometry
  emi_1349 : MinMax
  emi_1350 : Abs
  emi_{1353,1356..1357,1368} (4 alike) : Math  SaturateOnIntegerOverflow=on
  emi_1354 : Abs
  emi_1355 : Rounding
  emi_1358 : MinMax
  emi_1359 : Product  Inputs=*
  emi_1360 : Gain
  emi_1361 : Sin  TimeSource=Use external signal  SampleTime=0
  emi_1362 : Rounding
  emi_1363 : Sum  Inputs=+
  emi_1364 : Product  Inputs=*
  emi_1365 : Gain
  emi_1366 : Trigonometry
  emi_1367 : Gain
  emi_1369 : Rounding
  emi_1370 : UnaryMinus
  emi_1371 : Ground
  emi_1352 : Outport
  wires:
  emi_1351/1 -> emi_1348/1
  emi_1348/1 -> emi_1349/1
  emi_1349/1 -> emi_1350/1
  emi_1353/1 -> emi_1354/1
  emi_1354/1 -> emi_1355/1
  emi_1355/1 -> emi_1356/1
  emi_1356/1 -> emi_1357/1
  emi_1357/1 -> emi_1358/1
  emi_1358/1 -> emi_1359/1
  emi_1359/1 -> emi_1360/1
  emi_1360/1 -> emi_1361/1
  emi_1361/1 -> emi_1362/1
  emi_1362/1 -> emi_1363/1
  emi_1363/1 -> emi_1364/1
  emi_1364/1 -> emi_1365/1
  emi_1365/1 -> emi_1366/1
  emi_1366/1 -> emi_1367/1
  emi_1367/1 -> emi_1368/1
  emi_1368/1 -> emi_1369/1
  emi_1369/1 -> emi_1370/1
  emi_1371/1 -> emi_1353/1
  emi_1370/1 -> emi_1352/1

== system sampleModel646original/emi_1374 ==
  In1 : Inport
  emi_1375 : Inport  Port=2
  emi_1377 : Relay
  emi_1378 : Trigonometry
  emi_1379 : simulink/Discontinuities/Saturation Dynamic  OutMin=[]  OutMax=[]  OutDataTypeStr=Inherit: Same as second input  OutDataType=fixdt(1, 16)  OutScaling=2^-10  DoSatur=off
  emi_1380 : DiscreteFilter
  emi_1381 : Sin  TimeSource=Use external signal  SampleTime=0
  emi_1382 : DiscreteZeroPole  Poles=[0 0.5]  Gain=1  SampleTime=-1
  emi_1383 : UnaryMinus
  emi_1384 : Abs
  emi_1385 : DiscreteStateSpace  SampleTime=-1
  emi_1386 : slpidlib/PID Controller  Controller=PID  Form=Parallel  TimeDomain=Discrete-time  UseExternalTs=off  SampleTime=-1  IntegratorMethod=Forward Euler  FilterMethod=Forward Euler  ControllerParametersSource=internal  P=1  I=1  D=0  UseFilter=on  N=100  TunerSelectOption=Transfer Function Based (PID Tuner App)  InitialConditionSource=internal  InitialConditionForIntegrator=0  InitialConditionForFilter=0  DifferentiatorICPrevScaledInput=0  ExternalReset=none  TrackingMode=off  Kt=1  LimitOutput=off  SatLimitsSource=internal  UpperSaturationLimit=inf  LowerSaturationLimit=-inf  LinearizeAsGain=off  AntiWindupMode=none  Kb=1  POutMin=[]  POutMax=[]  IOutMin=[]  IOutMax=[]  DOutMin=[]  DOutMax=[]  NOutMin=[]  NOutMax=[]  SumOutMin=[]  SumOutMax=[]  SaturationOutMin=[]  SaturationOutMax=[]  PParamMin=[]  PParamMax=[]  IParamMin=[]  IParamMax=[]  DParamMin=[]  DParamMax=[]  NParamMin=[]  NParamMax=[]  KbParamMin=[]  KbParamMax=[]  KtParamMin=[]  KtParamMax=[]  KbOutMin=[]  KbOutMax=[]  KtOutMin=[]  KtOutMax=[]  IntegratorOutMin=[]  IntegratorOutMax=[]  FilterOutMin=[]  FilterOutMax=[]  SumI1OutMin=[]  SumI1OutMax=[]  SumI2OutMin=[]  SumI2OutMax=[]  SumI3OutMin=[]  SumI3OutMax=[]  SumI4OutMin=[]  SumI4OutMax=[]  SumDOutMin=[]  SumDOutMax=[]  DifferentiatorOutMin=[]  DifferentiatorOutMax=[]  FilterDiffOutCoefMin=[]  FilterDiffOutCoefMax=[]  ReciprocalOutMin=[]  ReciprocalOutMax=[]  SumDenOutMin=[]  SumDenOutMax=[]  SumNumOutMin=[]  SumNumOutMax=[]  DivideOutMin=[]  DivideOutMax=[]  UdiffTsProdOutMin=[]  UdiffTsProdOutMax=[]  NTsProdOutMin=[]  NTsProdOutMax=[]  UintegralTsProdOutMin=[]  UintegralTsProdOutMax=[]  UngainTsProdOutMin=[]  UngainTsProdOutMax=[]  IntegratorContinuousStateAttributes=''  IntegratorStateMustResolveToSignalObject=off  IntegratorRTWStateStorageClass=Auto  FilterContinuousStateAttributes=''  FilterStateMustResolveToSignalObject=off  FilterRTWStateStorageClass=Auto  ParallelPVariant=InternalParameters  IdealPVariant=Disabled  IVariant=InternalParameters  DVariant=InternalParameters  IntegratorVariant=Discrete  SatVariant=Disabled  AWVariant=Passthrough  PCopyVariant=Disabled  TRVariant=Disabled  FdbkBlocksVariant=Forward  IdealPFdbkVariant=Disabled  SatFdbkVariant=Disabled  DerivativeFilterVariant=ForwardEulerFilter  NVariant=InternalParameters  NCopyVariant=Disabled  FilterICVariant=InternalICsFilter  IntegratorICVariant=InternalICs  ExternalResetVariant=Disabled  TRSumVariant=Passthrough  SumFdbkVariant=Disabled  SumVariant=Sum_PID  TsampFilterVariant=InternalTs  TsampNgainVariant=Passthrough  TsampIntegralVariant=Passthrough  ExternalSaturationOutDataTypeStr=Inherit: Same as second input
  emi_1387 : DiscreteTransferFcn
  emi_1388 : Abs
  emi_1389 : DiscreteFilter
  emi_1390 : UnaryMinus
  emi_1391 : Clock
  Out1 : Outport
  emi_1376 : Outport  Port=2
  wires:
  In1/1 -> Out1/1
  emi_1377/1 -> emi_1378/1
  emi_1378/1 -> emi_1379/1
  emi_1379/1 -> emi_1380/1
  emi_1380/1 -> emi_1381/1
  emi_1381/1 -> emi_1382/1
  emi_1382/1 -> emi_1383/1
  emi_1383/1 -> emi_1384/1
  emi_1384/1 -> emi_1385/1
  emi_1385/1 -> emi_1386/1
  emi_1386/1 -> emi_1387/1
  emi_1387/1 -> emi_1388/1
  emi_1388/1 -> emi_1389/1
  emi_1389/1 -> emi_1390/1
  emi_1391/1 -> emi_1377/1
  emi_1390/1 -> emi_1376/1

== system sampleModel646original/emi_1399 ==
  emi_1406 : Inport
  Action Port : ActionPort  ActionPortLabel=if(0 > u1)
  emi_1403 : Abs
  emi_1404 : Math  SaturateOnIntegerOverflow=on
  emi_1405 : Trigonometry
  emi_1408 : Rounding
  emi_1409 : Ground
  emi_1407 : Outport
  wires:
  emi_1406/1 -> emi_1403/1
  emi_1403/1 -> emi_1404/1
  emi_1404/1 -> emi_1405/1
  emi_1409/1 -> emi_1408/1
  emi_1408/1 -> emi_1407/1

== system sampleModel646original/emi_1412 ==
  In1 : Inport
  emi_1413 : Inport  Port=2
  emi_1415 : DiscreteFir
  emi_1416 : Abs
  emi_1417 : DiscreteIntegrator  SampleTime=-1  ICPrevOutput=DiscIntNeverNeededParam  ICPrevScaledInput=DiscIntNeverNeededParam
  emi_1418 : Trigonometry
  emi_1419 : MinMax
  emi_1420 : Trigonometry
  emi_1421 : slpidlib/PID Controller  Controller=PID  Form=Parallel  TimeDomain=Discrete-time  UseExternalTs=off  SampleTime=-1  IntegratorMethod=Forward Euler  FilterMethod=Forward Euler  ControllerParametersSource=internal  P=1  I=1  D=0  UseFilter=on  N=100  TunerSelectOption=Transfer Function Based (PID Tuner App)  InitialConditionSource=internal  InitialConditionForIntegrator=0  InitialConditionForFilter=0  DifferentiatorICPrevScaledInput=0  ExternalReset=none  TrackingMode=off  Kt=1  LimitOutput=off  SatLimitsSource=internal  UpperSaturationLimit=inf  LowerSaturationLimit=-inf  LinearizeAsGain=off  AntiWindupMode=none  Kb=1  POutMin=[]  POutMax=[]  IOutMin=[]  IOutMax=[]  DOutMin=[]  DOutMax=[]  NOutMin=[]  NOutMax=[]  SumOutMin=[]  SumOutMax=[]  SaturationOutMin=[]  SaturationOutMax=[]  PParamMin=[]  PParamMax=[]  IParamMin=[]  IParamMax=[]  DParamMin=[]  DParamMax=[]  NParamMin=[]  NParamMax=[]  KbParamMin=[]  KbParamMax=[]  KtParamMin=[]  KtParamMax=[]  KbOutMin=[]  KbOutMax=[]  KtOutMin=[]  KtOutMax=[]  IntegratorOutMin=[]  IntegratorOutMax=[]  FilterOutMin=[]  FilterOutMax=[]  SumI1OutMin=[]  SumI1OutMax=[]  SumI2OutMin=[]  SumI2OutMax=[]  SumI3OutMin=[]  SumI3OutMax=[]  SumI4OutMin=[]  SumI4OutMax=[]  SumDOutMin=[]  SumDOutMax=[]  DifferentiatorOutMin=[]  DifferentiatorOutMax=[]  FilterDiffOutCoefMin=[]  FilterDiffOutCoefMax=[]  ReciprocalOutMin=[]  ReciprocalOutMax=[]  SumDenOutMin=[]  SumDenOutMax=[]  SumNumOutMin=[]  SumNumOutMax=[]  DivideOutMin=[]  DivideOutMax=[]  UdiffTsProdOutMin=[]  UdiffTsProdOutMax=[]  NTsProdOutMin=[]  NTsProdOutMax=[]  UintegralTsProdOutMin=[]  UintegralTsProdOutMax=[]  UngainTsProdOutMin=[]  UngainTsProdOutMax=[]  IntegratorContinuousStateAttributes=''  IntegratorStateMustResolveToSignalObject=off  IntegratorRTWStateStorageClass=Auto  FilterContinuousStateAttributes=''  FilterStateMustResolveToSignalObject=off  FilterRTWStateStorageClass=Auto  ParallelPVariant=InternalParameters  IdealPVariant=Disabled  IVariant=InternalParameters  DVariant=InternalParameters  IntegratorVariant=Discrete  SatVariant=Disabled  AWVariant=Passthrough  PCopyVariant=Disabled  TRVariant=Disabled  FdbkBlocksVariant=Forward  IdealPFdbkVariant=Disabled  SatFdbkVariant=Disabled  DerivativeFilterVariant=ForwardEulerFilter  NVariant=InternalParameters  NCopyVariant=Disabled  FilterICVariant=InternalICsFilter  IntegratorICVariant=InternalICs  ExternalResetVariant=Disabled  TRSumVariant=Passthrough  SumFdbkVariant=Disabled  SumVariant=Sum_PID  TsampFilterVariant=InternalTs  TsampNgainVariant=Passthrough  TsampIntegralVariant=Passthrough  ExternalSaturationOutDataTypeStr=Inherit: Same as second input
  emi_1422 : simulink/Discontinuities/Wrap To Zero  Threshold=255
      settings: SourceProductBaseCode=SL
  emi_1423 : simulink/Discontinuities/Rate Limiter Dynamic
  emi_1424 : DiscreteFilter
  emi_1425 : DiscreteFir
  emi_1426 : Sqrt  Operator=rSqrt  SaturateOnIntegerOverflow=on
  emi_1427 : DiscreteStateSpace  SampleTime=-1
  emi_1428 : DiscreteFir
  emi_1429 : simulink/Discrete/Transfer Fcn First Order  PoleZ=0.95  ICPrevOutput=0.0  DoSatur=off
  emi_1430 : DiscreteFilter
  emi_1431 : MinMax
  emi_1432 : simulink/Discontinuities/Saturation Dynamic  OutMin=[]  OutMax=[]  OutDataTypeStr=Inherit: Same as second input  OutDataType=fixdt(1, 16)  OutScaling=2^-10  DoSatur=off
  emi_1433 : DiscreteTransferFcn
  emi_1434 : DiscreteFilter
  emi_1435 : simulink/Discrete/Transfer Fcn First Order  PoleZ=0.95  ICPrevOutput=0.0  DoSatur=off
  emi_1436 : Gain
  emi_1437 : simulink/Discrete/Difference  ICPrevInput=0.0  OutMin=[]  OutMax=[]  OutDataType=fixdt(1, 16)  OutScaling=2^-10  DoSatur=off
  emi_1438 : simulink/Discontinuities/Rate Limiter Dynamic
  emi_1439 : Rounding
  emi_1440 : DigitalClock
  Out1 : Outport
  emi_1414 : Outport  Port=2
  wires:
  In1/1 -> Out1/1
  emi_1415/1 -> emi_1416/1
  emi_1416/1 -> emi_1417/1
  emi_1417/1 -> emi_1418/1
  emi_1418/1 -> emi_1419/1
  emi_1419/1 -> emi_1420/1
  emi_1420/1 -> emi_1421/1
  emi_1421/1 -> emi_1422/1
  emi_1422/1 -> emi_1423/1
  emi_1423/1 -> emi_1424/1
  emi_1424/1 -> emi_1425/1
  emi_1425/1 -> emi_1426/1
  emi_1426/1 -> emi_1427/1
  emi_1427/1 -> emi_1428/1
  emi_1428/1 -> emi_1429/1
  emi_1429/1 -> emi_1430/1
  emi_1430/1 -> emi_1431/1
  emi_1431/1 -> emi_1432/1
  emi_1432/1 -> emi_1433/1
  emi_1433/1 -> emi_1434/1
  emi_1434/1 -> emi_1435/1
  emi_1435/1 -> emi_1436/1
  emi_1436/1 -> emi_1437/1
  emi_1437/1 -> emi_1438/1
  emi_1438/1 -> emi_1439/1
  emi_1440/1 -> emi_1415/1
  emi_1439/1 -> emi_1414/1

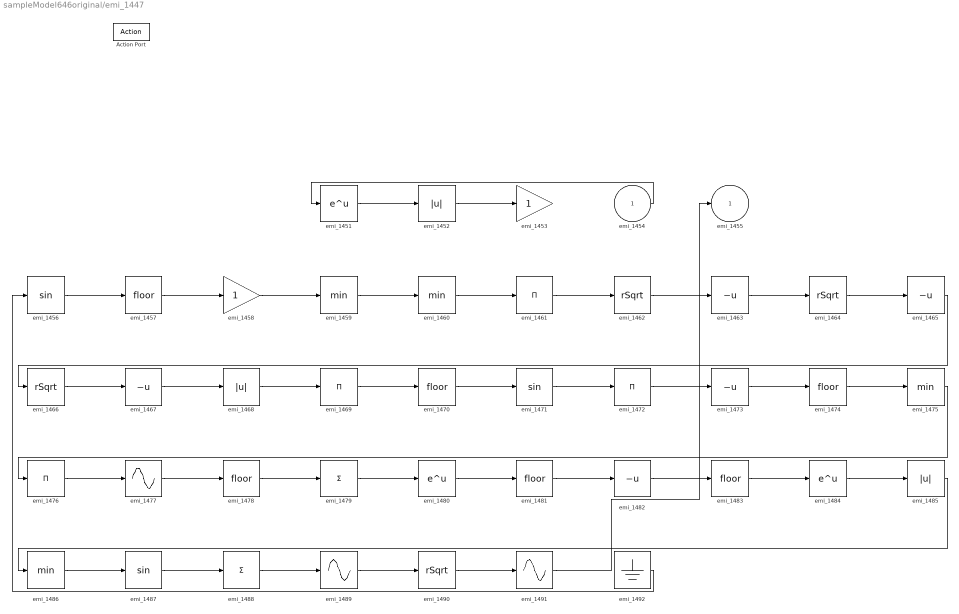
== system sampleModel646original/emi_1447 ==
  emi_1454 : Inport
  Action Port : ActionPort  ActionPortLabel=if(-1.617560e+02 > u1)
  emi_1451 : Math  SaturateOnIntegerOverflow=on
  emi_1452 : Abs
  emi_1453 : Gain
  emi_1456 : Trigonometry
  emi_{1457,1470,1474,1478,1481,1483} (6 alike) : Rounding
  emi_1458 : Gain
  emi_{1459..1460,1475,1486} (4 alike) : MinMax
  emi_{1461,1469,1472,1476} (4 alike) : Product  Inputs=*
  emi_{1462,1464,1466,1490} (4 alike) : Sqrt  Operator=rSqrt  SaturateOnIntegerOverflow=on
  emi_{1463,1465,1467,1473,1482} (5 alike) : UnaryMinus
  emi_1468 : Abs
  emi_1471 : Trigonometry
  emi_1477 : Sin  TimeSource=Use external signal  SampleTime=0
  emi_1479 : Sum  Inputs=+
  emi_1480 : Math  SaturateOnIntegerOverflow=on
  emi_1484 : Math  SaturateOnIntegerOverflow=on
  emi_1485 : Abs
  emi_1487 : Trigonometry
  emi_1488 : Sum  Inputs=+
  emi_1489 : Sin  TimeSource=Use external signal  SampleTime=0
  emi_1491 : Sin  TimeSource=Use external signal  SampleTime=0
  emi_1492 : Ground
  emi_1455 : Outport
  wires:
  emi_1454/1 -> emi_1451/1
  emi_1451/1 -> emi_1452/1
  emi_1452/1 -> emi_1453/1
  emi_1456/1 -> emi_1457/1
  emi_1457/1 -> emi_1458/1
  emi_1458/1 -> emi_1459/1
  emi_1459/1 -> emi_1460/1
  emi_1460/1 -> emi_1461/1
  emi_1461/1 -> emi_1462/1
  emi_1462/1 -> emi_1463/1
  emi_1463/1 -> emi_1464/1
  emi_1464/1 -> emi_1465/1
  emi_1465/1 -> emi_1466/1
  emi_1466/1 -> emi_1467/1
  emi_1467/1 -> emi_1468/1
  emi_1468/1 -> emi_1469/1
  emi_1469/1 -> emi_1470/1
  emi_1470/1 -> emi_1471/1
  emi_1471/1 -> emi_1472/1
  emi_1472/1 -> emi_1473/1
  emi_1473/1 -> emi_1474/1
  emi_1474/1 -> emi_1475/1
  emi_1475/1 -> emi_1476/1
  emi_1476/1 -> emi_1477/1
  emi_1477/1 -> emi_1478/1
  emi_1478/1 -> emi_1479/1
  emi_1479/1 -> emi_1480/1
  emi_1480/1 -> emi_1481/1
  emi_1481/1 -> emi_1482/1
  emi_1482/1 -> emi_1483/1
  emi_1483/1 -> emi_1484/1
  emi_1484/1 -> emi_1485/1
  emi_1485/1 -> emi_1486/1
  emi_1486/1 -> emi_1487/1
  emi_1487/1 -> emi_1488/1
  emi_1488/1 -> emi_1489/1
  emi_1489/1 -> emi_1490/1
  emi_1490/1 -> emi_1491/1
  emi_1492/1 -> emi_1456/1
  emi_1491/1 -> emi_1455/1

== system sampleModel646original/emi_1495 ==
  In1 : Inport
  emi_1496 : Inport  Port=2
  emi_1520 : Inport  Port=3  PortName=InBus  Element=signal1
  emi_1498 : Trigonometry
  emi_1499 : DiscreteStateSpace  SampleTime=-1
  emi_1500 : simulink/Discrete/Transfer Fcn First Order  PoleZ=0.95  ICPrevOutput=0.0  DoSatur=off
  emi_1501 : Math  SaturateOnIntegerOverflow=on
  emi_1502 : Trigonometry
  emi_1503 : simulink/Discrete/Discrete Derivative  gainval=1.0  ICPrevScaledInput=0.0  OutMin=[]  OutMax=[]  OutDataType=fixdt(1, 16)  OutScaling=2^-10  DoSatur=off
  emi_1504 : UnaryMinus
  emi_1505 : DiscreteZeroPole  Poles=[0 0.5]  Gain=1  SampleTime=-1
  emi_1506 : simulink/Discrete/Difference  ICPrevInput=0.0  OutMin=[]  OutMax=[]  OutDataType=fixdt(1, 16)  OutScaling=2^-10  DoSatur=off
  emi_1507 : Trigonometry
  emi_1508 : Math  SaturateOnIntegerOverflow=on
  emi_1509 : simulink/Discontinuities/Wrap To Zero  Threshold=255
      settings: SourceProductBaseCode=SL
  emi_1510 : Product  Inputs=*
  emi_1511 : simulink/Discrete/Difference  ICPrevInput=0.0  OutMin=[]  OutMax=[]  OutDataType=fixdt(1, 16)  OutScaling=2^-10  DoSatur=off
  emi_1512 : simulink/Discrete/Discrete Derivative  gainval=1.0  ICPrevScaledInput=0.0  OutMin=[]  OutMax=[]  OutDataType=fixdt(1, 16)  OutScaling=2^-10  DoSatur=off
  emi_1513 : simulink/Discrete/Difference  ICPrevInput=0.0  OutMin=[]  OutMax=[]  OutDataType=fixdt(1, 16)  OutScaling=2^-10  DoSatur=off
  emi_1514 : Quantizer
  emi_1515 : DiscreteIntegrator  SampleTime=-1  ICPrevOutput=DiscIntNeverNeededParam  ICPrevScaledInput=DiscIntNeverNeededParam
  emi_1516 : Abs
  emi_1517 : DiscreteStateSpace  SampleTime=-1
  emi_1518 : Sin  TimeSource=Use external signal  SampleTime=0
  emi_1519 : DiscreteTransferFcn
  Out1 : Outport
  emi_1497 : Outport  Port=2
  wires:
  In1/1 -> Out1/1
  emi_1498/1 -> emi_1499/1
  emi_1499/1 -> emi_1500/1
  emi_1500/1 -> emi_1501/1
  emi_1501/1 -> emi_1502/1
  emi_1502/1 -> emi_1503/1
  emi_1503/1 -> emi_1504/1
  emi_1504/1 -> emi_1505/1
  emi_1505/1 -> emi_1506/1
  emi_1506/1 -> emi_1507/1
  emi_1507/1 -> emi_1508/1
  emi_1508/1 -> emi_1509/1
  emi_1509/1 -> emi_1510/1
  emi_1510/1 -> emi_1511/1
  emi_1511/1 -> emi_1512/1
  emi_1512/1 -> emi_1513/1
  emi_1513/1 -> emi_1514/1
  emi_1514/1 -> emi_1515/1
  emi_1515/1 -> emi_1516/1
  emi_1516/1 -> emi_1517/1
  emi_1517/1 -> emi_1518/1
  emi_1518/1 -> emi_1519/1
  emi_1520/1 -> emi_1498/1
  emi_1519/1 -> emi_1497/1

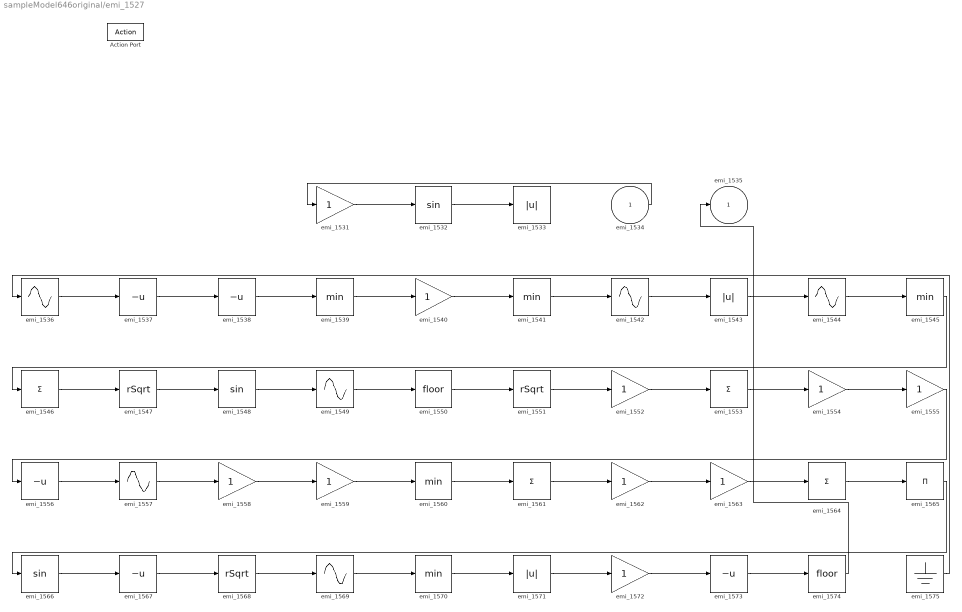
== system sampleModel646original/emi_1527 ==
  emi_1534 : Inport
  Action Port : ActionPort  ActionPortLabel=if(-1.617560e+02 > u1)
  emi_{1531,1540,1552,1554..1555,1558..1559,1562..1563,1572} (10 alike) : Gain
  emi_1532 : Trigonometry
  emi_1533 : Abs
  emi_{1536,1542,1544,1549,1557,1569} (6 alike) : Sin  TimeSource=Use external signal  SampleTime=0
  emi_{1537..1538,1556,1567,1573} (5 alike) : UnaryMinus
  emi_{1539,1541,1545,1560,1570} (5 alike) : MinMax
  emi_1543 : Abs
  emi_{1546,1553,1561,1564} (4 alike) : Sum  Inputs=+
  emi_1547 : Sqrt  Operator=rSqrt  SaturateOnIntegerOverflow=on
  emi_1548 : Trigonometry
  emi_1550 : Rounding
  emi_1551 : Sqrt  Operator=rSqrt  SaturateOnIntegerOverflow=on
  emi_1565 : Product  Inputs=*
  emi_1566 : Trigonometry
  emi_1568 : Sqrt  Operator=rSqrt  SaturateOnIntegerOverflow=on
  emi_1571 : Abs
  emi_1574 : Rounding
  emi_1575 : Ground
  emi_1535 : Outport
  wires:
  emi_1534/1 -> emi_1531/1
  emi_1531/1 -> emi_1532/1
  emi_1532/1 -> emi_1533/1
  emi_1536/1 -> emi_1537/1
  emi_1537/1 -> emi_1538/1
  emi_1538/1 -> emi_1539/1
  emi_1539/1 -> emi_1540/1
  emi_1540/1 -> emi_1541/1
  emi_1541/1 -> emi_1542/1
  emi_1542/1 -> emi_1543/1
  emi_1543/1 -> emi_1544/1
  emi_1544/1 -> emi_1545/1
  emi_1545/1 -> emi_1546/1
  emi_1546/1 -> emi_1547/1
  emi_1547/1 -> emi_1548/1
  emi_1548/1 -> emi_1549/1
  emi_1549/1 -> emi_1550/1
  emi_1550/1 -> emi_1551/1
  emi_1551/1 -> emi_1552/1
  emi_1552/1 -> emi_1553/1
  emi_1553/1 -> emi_1554/1
  emi_1554/1 -> emi_1555/1
  emi_1555/1 -> emi_1556/1
  emi_1556/1 -> emi_1557/1
  emi_1557/1 -> emi_1558/1
  emi_1558/1 -> emi_1559/1
  emi_1559/1 -> emi_1560/1
  emi_1560/1 -> emi_1561/1
  emi_1561/1 -> emi_1562/1
  emi_1562/1 -> emi_1563/1
  emi_1563/1 -> emi_1564/1
  emi_1564/1 -> emi_1565/1
  emi_1565/1 -> emi_1566/1
  emi_1566/1 -> emi_1567/1
  emi_1567/1 -> emi_1568/1
  emi_1568/1 -> emi_1569/1
  emi_1569/1 -> emi_1570/1
  emi_1570/1 -> emi_1571/1
  emi_1571/1 -> emi_1572/1
  emi_1572/1 -> emi_1573/1
  emi_1573/1 -> emi_1574/1
  emi_1575/1 -> emi_1536/1
  emi_1574/1 -> emi_1535/1
